simulink model "transcriptional_regulation_kalman_filter"  (R2021b)
settings: Solver=VariableStepAuto  StartTime=0.0  StopTime=10  RelTol=1e-3
undefined symbols (not defined in the file): As, Bs, control, Cs, K_pp, ki, Kp, kr_pp, L_k
libraries: simulink x1
settings Model: Creator=UTENTE  LastModifiedBy=UTENTE

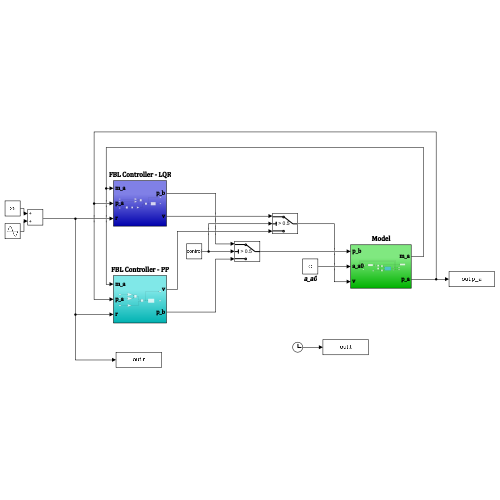
[thumbnail: Simulink's stored preview of the top-level diagram]
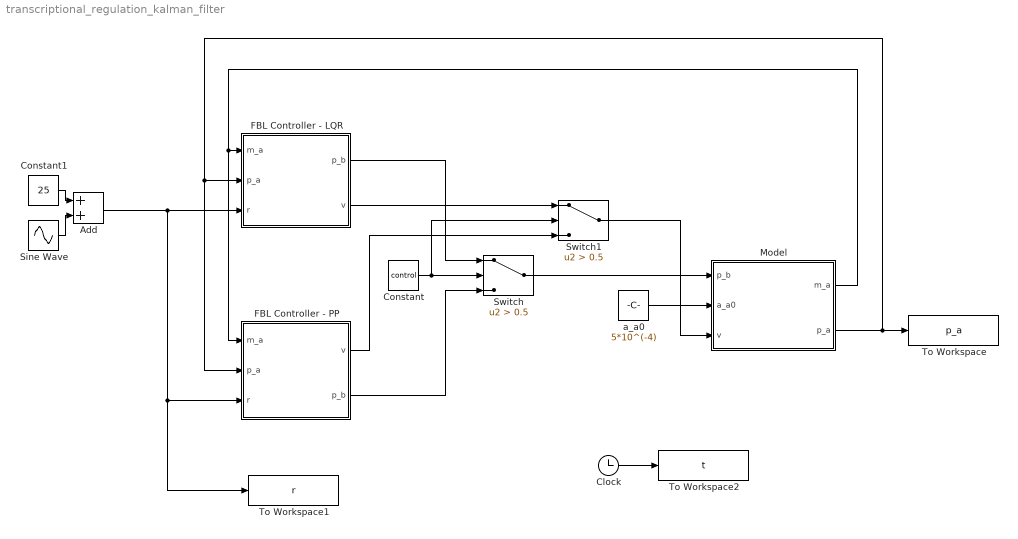
== system transcriptional_regulation_kalman_filter ==
  Add : Sum
  Clock : Clock
  Constant : Constant  Value=control
  Constant1 : Constant  Value=25
  FBL Controller - LQR : Subsystem
  FBL Controller - PP : Subsystem
  Model : Subsystem
  Sine Wave : Sin  Frequency=0.01  SampleTime=0
  Switch : Switch  Criteria=u2 > Threshold  Threshold=0.5
  Switch1 : Switch  Criteria=u2 > Threshold  Threshold=0.5
  To Workspace : ToWorkspace  VariableName=p_a  SampleTime=-1
  To Workspace1 : ToWorkspace  VariableName=r  SampleTime=-1
  To Workspace2 : ToWorkspace  VariableName=t  SampleTime=-1
  a_a0 : Constant  Value=5*10^(-4)
  wires:
  Add/1 -> FBL Controller - PP/3(r), To Workspace1/1, FBL Controller - LQR/3(r)
  a_a0/1 -> Model/2(a_a0)
  Clock/1 -> To Workspace2/1
  Constant1/1 -> Add/1
  Sine Wave/1 -> Add/2
  FBL Controller - LQR/1(p_b) -> Switch/1
  Constant/1 -> Switch1/2, Switch/2
  FBL Controller - PP/2(p_b) -> Switch/3
  Switch/1 -> Model/1(p_b)
  FBL Controller - LQR/2(v) -> Switch1/1
  FBL Controller - PP/1(v) -> Switch1/3
  Switch1/1 -> Model/3(v)
  Model/1(m_a) -> FBL Controller - PP/1(m_a), FBL Controller - LQR/1(m_a)
  Model/2(p_a) -> To Workspace/1, FBL Controller - PP/2(p_a), FBL Controller - LQR/2(p_a)

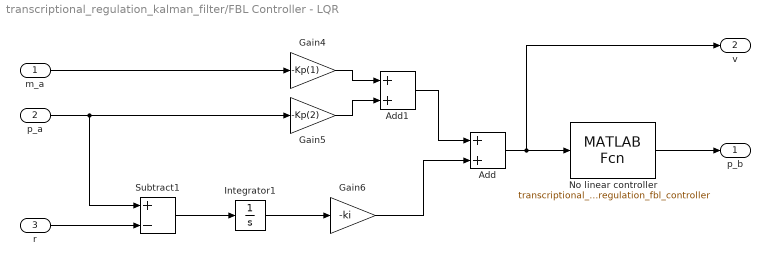
== system transcriptional_regulation_kalman_filter/FBL Controller - LQR ==
  m_a : Inport
  p_a : Inport  Port=2
  r : Inport  Port=3
  Add : Sum
  Add1 : Sum
  Gain4 : Gain  Gain=-Kp(1)
  Gain5 : Gain  Gain=-Kp(2)
  Gain6 : Gain  Gain=-ki
  Integrator1 : Integrator  InitialCondition=-30
  No linear controller : MATLABFcn  MATLABFcn=transcriptional_regulation_fbl_controller  OutputDimensions=1
  Subtract1 : Sum  Inputs=+-
  p_b : Outport
  v : Outport  Port=2
  wires:
  Integrator1/1 -> Gain6/1
  No linear controller/1 -> p_b/1
  m_a/1 -> Gain4/1
  Add1/1 -> Add/1
  r/1 -> Subtract1/2
  Gain6/1 -> Add/2
  Add/1 -> v/1, No linear controller/1
  Gain4/1 -> Add1/1
  p_a/1 -> Gain5/1, Subtract1/1
  Gain5/1 -> Add1/2
  Subtract1/1 -> Integrator1/1

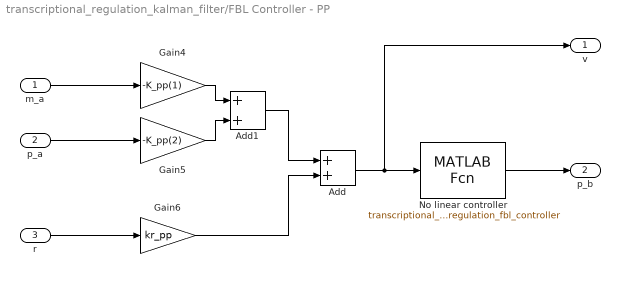
== system transcriptional_regulation_kalman_filter/FBL Controller - PP ==
  m_a : Inport
  p_a : Inport  Port=2
  r : Inport  Port=3
  Add : Sum
  Add1 : Sum
  Gain4 : Gain  Gain=-K_pp(1)
  Gain5 : Gain  Gain=-K_pp(2)
  Gain6 : Gain  Gain=kr_pp
  No linear controller : MATLABFcn  MATLABFcn=transcriptional_regulation_fbl_controller  OutputDimensions=1
  v : Outport
  p_b : Outport  Port=2
  wires:
  Gain5/1 -> Add1/2
  p_a/1 -> Gain5/1
  Gain4/1 -> Add1/1
  Gain6/1 -> Add/2
  r/1 -> Gain6/1
  Add1/1 -> Add/1
  m_a/1 -> Gain4/1
  No linear controller/1 -> p_b/1
  Add/1 -> v/1, No linear controller/1

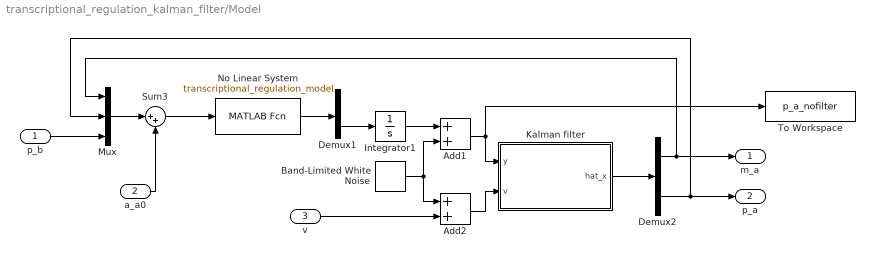
== system transcriptional_regulation_kalman_filter/Model ==
  p_b : Inport
  a_a0 : Inport  Port=2
  v : Inport  Port=3
  Add1 : Sum
  Add2 : Sum
  Band-Limited White Noise : simulink/Sources/Band-Limited White Noise  Cov=[0.1]  Ts=0.1  seed=[23341]
  Demux1 : Demux  Outputs=2
  Demux2 : Demux  Outputs=2
  Integrator1 : Integrator  InitialCondition=30
  Kalman filter : Subsystem
  Mux : Mux  Inputs=3
  No Linear System : MATLABFcn  MATLABFcn=transcriptional_regulation_model  OutputDimensions=2
  Sum3 : Sum  Inputs=|++
  To Workspace : ToWorkspace  VariableName=p_a_nofilter  SampleTime=-1
  m_a : Outport
  p_a : Outport  Port=2
  wires:
  Sum3/1 -> No Linear System/1
  No Linear System/1 -> Demux1/1
  Mux/1 -> Sum3/1
  a_a0/1 -> Sum3/2
  Demux1/2 -> Integrator1/1
  Integrator1/1 -> Add1/1
  p_b/1 -> Mux/3
  Kalman filter/1(hat_x) -> Demux2/1
  Demux2/1 -> Mux/1, m_a/1
  Demux2/2 -> p_a/1, Mux/2
  v/1 -> Add2/2
  Add1/1 -> Kalman filter/1(y), To Workspace/1
  Add2/1 -> Kalman filter/2(v)
  Band-Limited White Noise/1 -> Add1/2, Add2/1

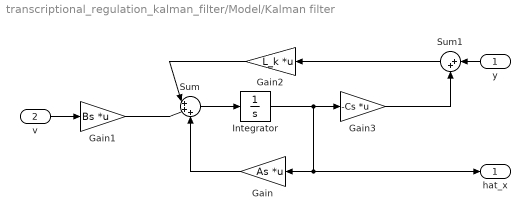
== system transcriptional_regulation_kalman_filter/Model/Kalman filter ==
  y : Inport
  v : Inport  Port=2
  Gain : Gain  Gain=As  Multiplication=Matrix(K*u)
  Gain1 : Gain  Gain=Bs  Multiplication=Matrix(K*u)
  Gain2 : Gain  Gain=L_k  Multiplication=Matrix(K*u)
  Gain3 : Gain  Gain=-Cs  Multiplication=Matrix(K*u)
  Integrator : Integrator  InitialCondition=30
  Sum : Sum  Inputs=|+++
  Sum1 : Sum  Inputs=|++
  hat_x : Outport
  wires:
  Sum/1 -> Integrator/1
  Gain2/1 -> Sum/1
  Gain3/1 -> Sum1/2
  y/1 -> Sum1/1
  Integrator/1 -> Gain/1, hat_x/1, Gain3/1
  Gain1/1 -> Sum/2
  Sum1/1 -> Gain2/1
  Gain/1 -> Sum/3
  v/1 -> Gain1/1
